simulink model "test_power_pll"  (R2018b)
settings: Solver=FixedStepAuto  StartTime=0.0  StopTime=35  FixedStep=0.00075  RelTol=1e-3
undefined symbols (not defined in the file): DiscIntNeverNeededParam
libraries: simulink x4
settings Model: Creator=dengzhe  LastModifiedBy=dengzhe

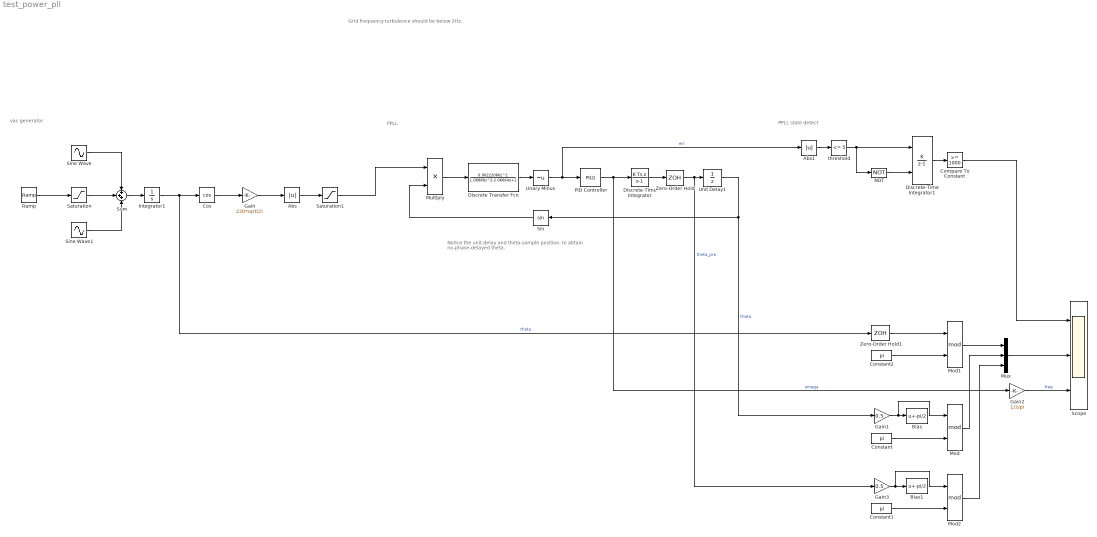
== system test_power_pll ==
  note: PPLL state detect
  note: Notice the unit-delay and theta-sample position,
      | to abtain no-phase-delayed theta.
  note: Grid frequency turbulence should be below 2Hz.
  note: PPLL
  note: vac generator
  Abs : Abs
  Abs1 : Abs
  Bias : Bias  Bias=-pi/2
  Bias1 : Bias  Bias=-pi/2
  Compare To Constant : simulink/Logic and Bit Operations/Compare To Constant  relop=>=  const=1000  OutDataTypeStr=boolean
  Constant : Constant  Value=pi
  Constant1 : Constant  Value=pi
  Constant2 : Constant  Value=pi
  Cos : Trigonometry  Operator=cos
  Discrete Transfer Fcn : DiscreteTransferFcn  Numerator=[0.00222066 0 0]  Denominator=[1.06886 -2.06664 1]
  Discrete-Time Integrator : DiscreteIntegrator  IntegratorMethod=Integration: Backward Euler  SampleTime=-1  ICPrevOutput=DiscIntNeverNeededParam  ICPrevScaledInput=DiscIntNeverNeededParam
  Discrete-Time Integrator1 : DiscreteIntegrator  IntegratorMethod=Accumulation: Forward Euler  ExternalReset=level  SampleTime=-1  OutDataTypeStr=double  LimitOutput=on  UpperSaturationLimit=1000  LowerSaturationLimit=0  ICPrevOutput=DiscIntNeverNeededParam  ICPrevScaledInput=DiscIntNeverNeededParam
  Gain : Gain  Gain=220*sqrt(2)
  Gain1 : Gain  Gain=0.5
  Gain2 : Gain  Gain=1/2/pi
  Gain3 : Gain  Gain=0.5
  Integrator1 : Integrator  InitialCondition=0.5
  Mod : Math  Operator=mod  SaturateOnIntegerOverflow=on
  Mod1 : Math  Operator=mod  SaturateOnIntegerOverflow=on
  Mod2 : Math  Operator=mod  SaturateOnIntegerOverflow=on
  Multiply : Product
  Mux : Mux  Inputs=3
  NOT : Logic  Operator=NOT  AllPortsSameDT=off  OutDataTypeStr=boolean
  PID Controller : simulink/Continuous/PID Controller  Controller=PI  Form=Parallel  TimeDomain=Discrete-time  SampleTime=-1  IntegratorMethod=Backward Euler  FilterMethod=Forward Euler  ControllerParametersSource=internal  P=0.1  I=2  D=0  UseFilter=on  N=100  TunerSelectOption=Transfer Function Based (PID Tuner App)  InitialConditionSource=internal  InitialConditionForIntegrator=2*pi*100  InitialConditionForFilter=0  DifferentiatorICPrevScaledInput=0  ExternalReset=none  TrackingMode=off  Kt=1  LimitOutput=on  UpperSaturationLimit=2*pi*140  LowerSaturationLimit=2*pi*80  LinearizeAsGain=on  AntiWindupMode=clamping  Kb=1  POutMin=[]  POutMax=[]  IOutMin=[]  IOutMax=[]  DOutMin=[]  DOutMax=[]  NOutMin=[]  NOutMax=[]  SumOutMin=[]  SumOutMax=[]  SaturationOutMin=[]  SaturationOutMax=[]  PParamMin=[]  PParamMax=[]  IParamMin=[]  IParamMax=[]  DParamMin=[]  DParamMax=[]  NParamMin=[]  NParamMax=[]  KbParamMin=[]  KbParamMax=[]  KtParamMin=[]  KtParamMax=[]  KbOutMin=[]  KbOutMax=[]  KtOutMin=[]  KtOutMax=[]  IntegratorOutMin=[]  IntegratorOutMax=[]  FilterOutMin=[]  FilterOutMax=[]  SumI1OutMin=[]  SumI1OutMax=[]  SumI2OutMin=[]  SumI2OutMax=[]  SumI3OutMin=[]  SumI3OutMax=[]  SumI4OutMin=[]  SumI4OutMax=[]  SumDOutMin=[]  SumDOutMax=[]  DifferentiatorOutMin=[]  DifferentiatorOutMax=[]  FilterDiffOutCoefMin=[]  FilterDiffOutCoefMax=[]  ReciprocalOutMin=[]  ReciprocalOutMax=[]  SumDenOutMin=[]  SumDenOutMax=[]  SumNumOutMin=[]  SumNumOutMax=[]  DivideOutMin=[]  DivideOutMax=[]  IntegratorContinuousStateAttributes=''  IntegratorStateMustResolveToSignalObject=off  IntegratorRTWStateStorageClass=Auto  FilterContinuousStateAttributes=''  FilterStateMustResolveToSignalObject=off  FilterRTWStateStorageClass=Auto  ParallelPVariant=InternalParameters  IdealPVariant=Disabled  IVariant=InternalParameters  DVariant=Disabled  IntegratorVariant=Discrete  SatVariant=Enabled  AWVariant=DiscClampingParallel  PCopyVariant=Disabled  TRVariant=Disabled  FdbkBlocksVariant=Feedback  IdealPFdbkVariant=Passthrough  SatFdbkVariant=Passthrough  DerivativeFilterVariant=Disabled  NVariant=Disabled  NCopyVariant=Disabled_SignalSpec  FilterICVariant=Disabled  IntegratorICVariant=InternalICs  ExternalResetVariant=Disabled  TRSumVariant=Passthrough  SumFdbkVariant=Enabled  SumVariant=Sum_PI
  Ramp : simulink/Sources/Ramp  slope=2*pi*5/5  start=5  InitialOutput=2*pi*48
  Saturation : Saturate  UpperLimit=2*pi*65  LowerLimit=0
  Saturation1 : Saturate  UpperLimit=inf  LowerLimit=50
      settings: AttributesFormatString=lower limit: %<LowerLimit>
  Scope : Scope  NumInputPorts=3
  Sin : Trigonometry
  Sine Wave : Sin  Amplitude=2*pi*1  Frequency=2*pi*100  SampleTime=0
  Sine Wave1 : Sin  Amplitude=2*pi*1  Frequency=2*pi*173  SampleTime=0
  Sum : Sum  Inputs=+++
  Unary Minus : UnaryMinus
  Unit Delay1 : UnitDelay  InitialCondition=2*pi*100  SampleTime=-1
  Zero-Order Hold : ZeroOrderHold  SampleTime=-1
  Zero-Order Hold1 : ZeroOrderHold  SampleTime=-1
  threshold : simulink/Logic and Bit Operations/Compare To Constant  relop=<=  const=5  OutDataTypeStr=boolean
  wires:
  Cos/1 -> Gain/1
  Discrete-Time Integrator/1 -> Zero-Order Hold/1
  Multiply/1 -> Discrete Transfer Fcn/1
  Gain/1 -> Abs/1
  Constant/1 -> Mod/2
  Mod/1 -> Mux/2
  Integrator1/1 -> Zero-Order Hold1/1, Cos/1  "theta"
  Ramp/1 -> Saturation/1
  Constant2/1 -> Mod1/2
  Mod1/1 -> Mux/1
  Zero-Order Hold1/1 -> Mod1/1
  Mux/1 -> Scope/2
  Gain2/1 -> Scope/3  "freq"
  PID Controller/1 -> Discrete-Time Integrator/1, Gain2/1  "omega"
  Abs/1 -> Saturation1/1
  Saturation/1 -> Sum/2
  Unary Minus/1 -> Abs1/1, PID Controller/1  "err"
  Sine Wave/1 -> Sum/1
  Sine Wave1/1 -> Sum/3
  Saturation1/1 -> Multiply/1
  Sum/1 -> Integrator1/1
  Unit Delay1/1 -> Sin/1, Gain1/1  "theta"
  Zero-Order Hold/1 -> Gain3/1, Unit Delay1/1  "theta_pre"
  Gain3/1 -> Mod2/1, Bias1/1
  Mod2/1 -> Mux/3
  Constant1/1 -> Mod2/2
  Abs1/1 -> threshold/1
  NOT/1 -> Discrete-Time Integrator1/2
  Discrete-Time Integrator1/1 -> Compare To Constant/1
  threshold/1 -> Discrete-Time Integrator1/1, NOT/1
  Compare To Constant/1 -> Scope/1
  Gain1/1 -> Mod/1, Bias/1
  Sin/1 -> Multiply/2
  Discrete Transfer Fcn/1 -> Unary Minus/1
